simulink model "power_turbine"  (Simulink 6.0)
settings: Solver=ode23tb  SolverMode=SingleTasking  StartTime=0.0  StopTime=2  RelTol=1e-3
undefined symbols (not defined in the file or in its folder): D1, Delta
libraries: powerlib x11
settings Model: Creator=patrice  LastModifiedBy=batserve  ExtModeTrigMode=oneshot  ExtModeArmWhenConnect=off  ExtModeAutoUpdateStatusClock=off
settings DataIOCC: LimitDataPoints=off  SignalLoggingName=sigsOut
settings OptimizationCC: BlockReduction=off  BooleanDataType=off
settings DebuggingCC: CheckExecutionContextPreStartOutputMsg=on  CheckExecutionContextRuntimeOutputMsg=on  SolverPrmCheckMsg=none
settings HardwareCC: TargetUnknown=on
settings RTWCC: TemplateMakefile=grt_unix.tmf

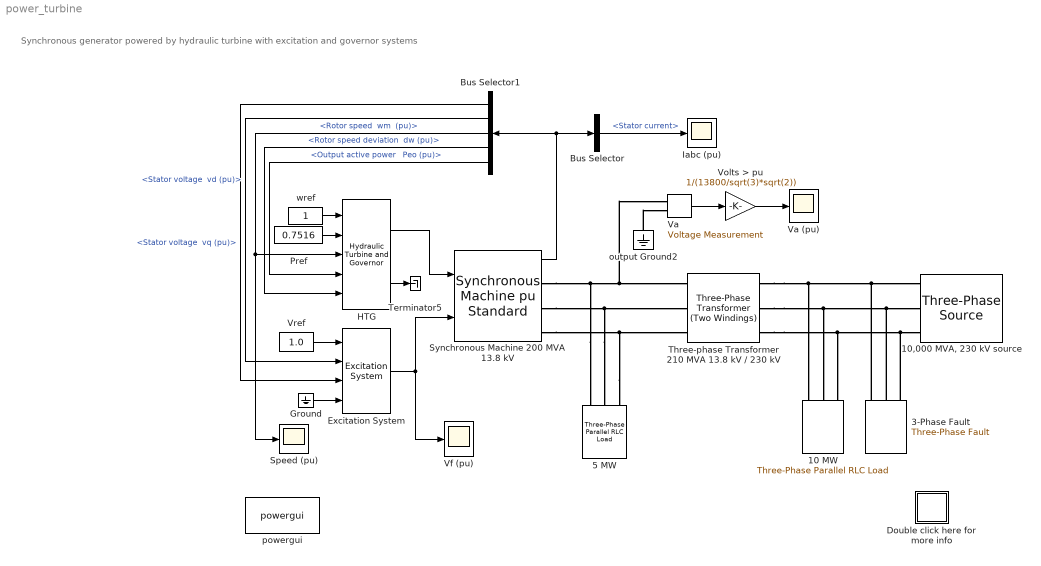
== system power_turbine ==
  note: Synchronous generator powered by hydraulic turbine
      |  with excitation and governor systems
  " Iabc (pu)" : Scope
      settings: TickLabels=on  TimeRange=0.2  YMax=6  DataFormat=Array
  " Speed (pu)" : Scope
      settings: TickLabels=on  TimeRange=2  YMin=0.98  YMax=1.02  SaveName=Pm  DataFormat=Array
  10 MW : powerlib/Elements/Three-Phase Parallel RLC Load  Orientation=down  PhysicalDomain=powersysdomain  SubClassName=unknown  LeftPortType=p1  RightPortType=p1  LConnTagsString=A|B|C  Configuration=Y (grounded)  NominalVoltage=230e3  NominalFrequency=60  ActivePower=10e6  InductivePower=0  CapacitivePower=0  Measurements=None
  "10,000 MVA, 230 kV source" : powerlib/Electrical Sources/Three-Phase Source  Orientation=left  Voltage=230e3  PhaseAngle=0  Frequency=60  InternalConnection=Yg  SpecifyImpedance=on  Resistance=0.529  Inductance=0.0140  ShortCircuitLevel=10000e6  BaseVoltage=230e3  XRratio=10
  3-Phase Fault : powerlib/Elements/Three-Phase Fault  Orientation=down  FaultA=on  FaultB=on  FaultC=on  FaultResistance=1e-3  GroundFault=on  GroundResistance=1e-3  External=off  SwitchStatus=[1 0]  SwitchTimes=[ 0.1 0.2]  InitialStates=[1 1 0]  SnubberResistance=inf  SnubberCapacitance=inf  Measurements=None
  5 MW : powerlib/Elements/Three-Phase Parallel RLC Load  Orientation=down  PhysicalDomain=powersysdomain  SubClassName=unknown  LeftPortType=p1  RightPortType=p1  LConnTagsString=A|B|C  Configuration=Y (grounded)  NominalVoltage=13.8e3  NominalFrequency=60  ActivePower=5e6  InductivePower=0  CapacitivePower=0  Measurements=None
  Bus Selector : BusSelector  DialogController=Simulink.DDGSource_Bus  OutputSignals=Stator current
  Bus Selector1 : BusSelector  Orientation=left  DialogController=Simulink.DDGSource_Bus  OutputSignals="dq0 components.Stator voltage  vq (pu),dq0 components.Stator voltage  vd (pu),Mechanical.Rotor speed  wm  (pu),Mechanical.Rotor speed deviation  dw (pu),Output active power   Peo (pu)"
  Double click here for more info : Subsystem
      mask Display: disp('?')
  Excitation System : powerlib/Machines/Excitation System  tr=20e-3  reg=[ 300, 0.001 ]  exc=[ 1, 0 ]  tgr=[ 0, 0 ]  damp=[ 0.001, 0.1 ]  sat=[ 0, 0 ]  lim=[ -11.5, 11.5, 0 ]  v0=[1,1.0]
  Ground : Ground
  HTG : powerlib/Machines/Hydraulic Turbine and Governor  sm="[ 10/3  0.07 ]"  gate="[  0.01  0.97518  -0.1  0.1 ]"  reg="[  0.05  1.163  0.105  0  0.01  ]"  hyd="[  0  2.67  ]"  dref=0  po=1
  Pref : Constant  Value=0.7516
  Synchronous Machine 200 MVA 13.8 kV : powerlib/Machines/Synchronous Machine pu Standard  PresetModel=No  ShowDetailedParameters=on  RotorType=Salient-pole  NominalParameters="[ 200E6  13800   60 ]"  Reactances1=[ 31 32 33 34 35 36 37 ]  Reactances2=[ 1.305, 0.296, 0.252, 0.474, 0.243, 0.18 ]  dAxisTimeConstants=Short-circuit  qAxisTimeConstants=Open-circuit  TimeConstants1=[]  TimeConstants2=[]  TimeConstants3=[]  TimeConstants4=[]  TimeConstants5=[ 1.01, 0.053, 0.1 ]  TimeConstants6=[]  TimeConstants7=[]  TimeConstants8=[]  StatorResistance=2.8544e-3  Mechanical="[ 3.2 0  32]"  InitialConditions=[0 0 0 0 0 0 0 0 1]  SetSaturation=off  Saturation=[0.6404,0.7127,0.8441,0.9214,0.9956,1.082,1.19,1.316,1.457;0.7,0.7698,0.8872,0.9466,0.9969,1.046,1.1,1.151,1.201]  Units=0.5  LoadFlowParameters=[1 150000000 0 0]
      settings: AttributesFormatString=\n\n
  Terminator5 : Terminator
  Three-phase Transformer 210 MVA 13.8 kV / 230 kV : powerlib/Elements/Three-Phase Transformer (Two Windings)  NominalPower=[ 210e6 60 ]  Winding1Connection=Delta (D1)  Winding1="[ 13.8e3 0.0027  0.08]"  Winding2Connection=Yg  Winding2=[ 230e3 0.0027 0.08]  SetSaturation=off  Rm=500  Lm=500  Saturation="[ 0,0  ;  0.005,1.2  ;  1.0,1.4 ]"  Hysteresis=off  DataFile='hysteresis'  SetInitialFlux=off  InitialFluxes=[ 0.8 , -0.8 , 0.7 ]  Measurements=None  TransfoNumber=0
  Va : powerlib/Measurements/Voltage Measurement  Tag=PoWeRsYsTeMmEaSuReMeNt  PhasorSimulation=off  OutputType=Magnitude  PSBequivalent=0
  Va (pu) : Scope
      settings: TickLabels=on  TimeRange=0.2  YMin=-1.25  YMax=1.25  SaveName=vf  DataFormat=Array
  Vf (pu) : Scope
      settings: TickLabels=on  TimeRange=2  YMin=-10  YMax=15  SaveName=vf  DataFormat=Array
  Volts > pu : Gain  Gain=1/(13800/sqrt(3)*sqrt(2))  SaturateOnIntegerOverflow=on
  Vref : Constant  Value=1.0
  output Ground2 : powerlib/Elements/Ground  Orientation=down  PhysicalDomain=powersysdomain  SubClassName=unknown  LeftPortType=p1  RightPortType=p1  LConnTagsString=a
  powergui : powerlib/powergui  Priority=2  Frange=logspace(0,3,50)  Ylog=off  Xlog=off  save=off  variable=ZData  ZoomFFT=on  StartTime=0.0  cycles=2  DisplayStyle=off  fundamental=60  FreqAxis=off  MaxFrequency=1000  frequencyindice=60  frequencyindicesteady=1  RmsSteady=1  display=off  Ts=0  methode=off  frequency=60  echomessages=on
  wref : Constant
  wires:
  Ground/1 -> Excitation System/4
  HTG/2 -> Terminator5/1
  Vref/1 -> Excitation System/1
  Pref/1 -> HTG/2
  wref/1 -> HTG/1
  Volts > pu/1 -> Va (pu)/1
  Excitation System/1 -> Vf (pu)/1, Synchronous Machine 200 MVA 13.8 kV/2
  HTG/1 -> Synchronous Machine 200 MVA 13.8 kV/1
  Synchronous Machine 200 MVA 13.8 kV/1 -> Bus Selector/1, Bus Selector1/1
  Va/1 -> Volts > pu/1
  Bus Selector/1 -> " Iabc (pu)"/1  "<Stator current>"
  Bus Selector1/1 -> Excitation System/3  "<Stator voltage  vq (pu)>"
  Bus Selector1/2 -> Excitation System/2  "<Stator voltage  vd (pu)>"
  Bus Selector1/3 -> HTG/3, " Speed (pu)"/1  "<Rotor speed  wm  (pu)>"
  Bus Selector1/4 -> HTG/5  "<Rotor speed deviation  dw (pu)>"
  Bus Selector1/5 -> HTG/4  "<Output active power   Peo (pu)>"
  connections:
  output Ground2/LConn1 -- Va/LConn2
  Synchronous Machine 200 MVA 13.8 kV/RConn3 -- 5 MW/LConn3 -- Three-phase Transformer 210 MVA 13.8 kV / 230 kV/LConn3
  Synchronous Machine 200 MVA 13.8 kV/RConn2 -- 5 MW/LConn2 -- Three-phase Transformer 210 MVA 13.8 kV / 230 kV/LConn2
  Synchronous Machine 200 MVA 13.8 kV/RConn1 -- Va/LConn1 -- Three-phase Transformer 210 MVA 13.8 kV / 230 kV/LConn1 -- 5 MW/LConn1
  Three-phase Transformer 210 MVA 13.8 kV / 230 kV/RConn1 -- 3-Phase Fault/LConn1 -- "10,000 MVA, 230 kV source"/RConn1 -- 10 MW/LConn1
  Three-phase Transformer 210 MVA 13.8 kV / 230 kV/RConn2 -- 3-Phase Fault/LConn2 -- "10,000 MVA, 230 kV source"/RConn2 -- 10 MW/LConn2
  Three-phase Transformer 210 MVA 13.8 kV / 230 kV/RConn3 -- 3-Phase Fault/LConn3 -- "10,000 MVA, 230 kV source"/RConn3 -- 10 MW/LConn3

== system power_turbine/Double click here for more info ==
  note: 4
  note: In order to start the simulation in steady state with the HTG and excitation system connected,  these two Simulink blocks must also be initialized
      | according to the values calculated by the load flow. This initialization is automatically performed when you execute the Load Flow, as long as you connect  at
      | the Pm and Vf inputs of the machine either Constant blocks or regulation blocks from the machine library (HTG, STG, or Excitation System).
      | Open the HTG block menu and notice that the initial mechanical  power has been automatically set to 0.5007 pu (100.14 MW) by the Load Flow.
      | Then, open the Excitation System block menu and note that the initial terminal voltage and field voltage have been set respectively to 1.0 and 1.1291 pu.
  note: 2
  note: Start Simulation and observe the three machine currents on the Iabc scope. If  the 9 parameters defining initial conditions
      | for the Synchronous Machine are set at zero or not set correctly, the simulation will not start in steady state.
  note: A three-phase generator rated 200 MVA, 13.8 kV, 112.5 rpm is connected to a 230 kV, 10,000 MVA network through a Delta-Wye 210 MVA transformer.
      | At t = 0.1 s, a three-phase to ground fault occurs on the 230 kV bus. The fault is cleared after 6 cycles (t = 0.2 s).
      | During this demo, you will initialize the system in order to start in steady-state with the generator  supplying 150 MW of active power
      | and observe the dynamic response of the machine and of its voltage and speed regulators.
  note: This demonstration illustrates use of the synchronous machine associated with
      | the Hydraulic Turbine and Governor (HTG) and Excitation System blocks and use of
      | the Load Flow to initialize machine currents
  note: Circuit Description
  note: Demonstration
  note: 1
  note: 3
  note: Open the 4 scopes and restart the simulation. The simulation now starts in steady state.
      | Observe that the terminal voltage Va is 1.0 p.u. at the beginning of the simulation. It falls to about 0.4 pu during the fault and returns to nominal
      | quickly after the fault is cleared. This quick response in terminal voltage is due to the fact that the Excitation System output Vf can go as high as 11.5 pu
      | which it does during the fault. The speed of the machine  increases to 1.01 pu during the fault then  it oscillates around 1 p.u. as the governor system regulates it.
      | The speed takes much longer than the terminal voltage to stabilize mainly because the rate of valve opening/closing in the governor system is limited to 0.1 pu/s.
  note: In order to start the simulation in steady-state you must initialize the synchronous machine for the desired load flow.
      | Open the Powergui and select 'Load Flow and Machine Initialization' . A new window appears. The machine 'Bus type' should be already initialized as
      | 'PV generator', indicating that  the load flow will be performed with the machine controlling the active power and its terminal voltage.
      | Specify the desired values by entering  the following parameters :
  note: Louis-A. Dessaint and R. Champagne (Ecole de Technologie Superieure, Montreal)
  note: Once the load flow has been solved the phasors of AB and BC machine voltages as well as the currents flowing out of phases A and B are updated.
      | The machine reactive power,  mechanical power and  field voltage requested to supply the electrical power should also be displayed:
      | Q = 3.4 Mvar; Pmec = 150.32 MW (0.7516 pu); field voltage Ef = 1.291 pu.
  note: Load flow : Terminal voltage (Vrms) = 13800; Active Power = 150e6. Then press the 'Execute Load Flow' button.
